simulink model "Aktuator_Klapp"  (R2019b)
settings: Solver=FixedStepAuto  StartTime=0.0  StopTime=9  RelTol=1e-3
values from neighbouring files (symbols this model uses):
  a = 0.047    [Init_Aktuator_Klapp.m]
  Drehzahlkonstante = 1070    [Init_Aktuator.m]    (also in Init_Aktuator_Klapp.m = 569; Init_Aktuator_Steuer.m)
  I_GF = 0.16    [Init_Aktuator_Klapp.m]
  I_Konstante = 20    [Init_Aktuator.m]    (also in Init_Aktuator_Steuer.m)
  I_Motor = 0.0000132    (= 1.32e-05)    [Init_Aktuator_Klapp.m]
  I_Spindel = 0    [Init_Aktuator_Klapp.m]
  Kennliniensteigung = 108*1000    (= 108000)    [Init_Aktuator_Klapp.m]
  M_Hubstange = 0.02    [Init_Aktuator_Klapp.m]
  P_Konstante = 4    [Init_Aktuator.m]    (also in Init_Aktuator_Steuer.m)
  r = 0.016    [Init_Aktuator_Klapp.m]
  Reibungsbeiwert = 0.0018    [Init_Aktuator_Steuer.m]
  Spannung = 12    [Init_Aktuator_Klapp.m]
  Spannung_max = Nennspannung * 2    (= 24)    [Init_Aktuator.m]    (also in Init_Aktuator_Steuer.m = 18)
  Steigung = 27.1*1000    (= 27100)    [Init_Aktuator.m]    (also in Init_Aktuator_Klapp.m = 0.002; Init_Aktuator_Steuer.m)
  Uebersetzung = 200    [Init_Aktuator.m]    (also in Init_Aktuator_Klapp.m = 3.7; Init_Aktuator_Steuer.m)
undefined symbols (not defined in the file or in its folder): Hebelarm, Normalkraft, Wirkungsgrad
libraries: simulink x1
settings Model: Creator=Neu1  LastModifiedBy=Neu1
settings SolverCC: AlgebraicLoopSolver=LineSearch

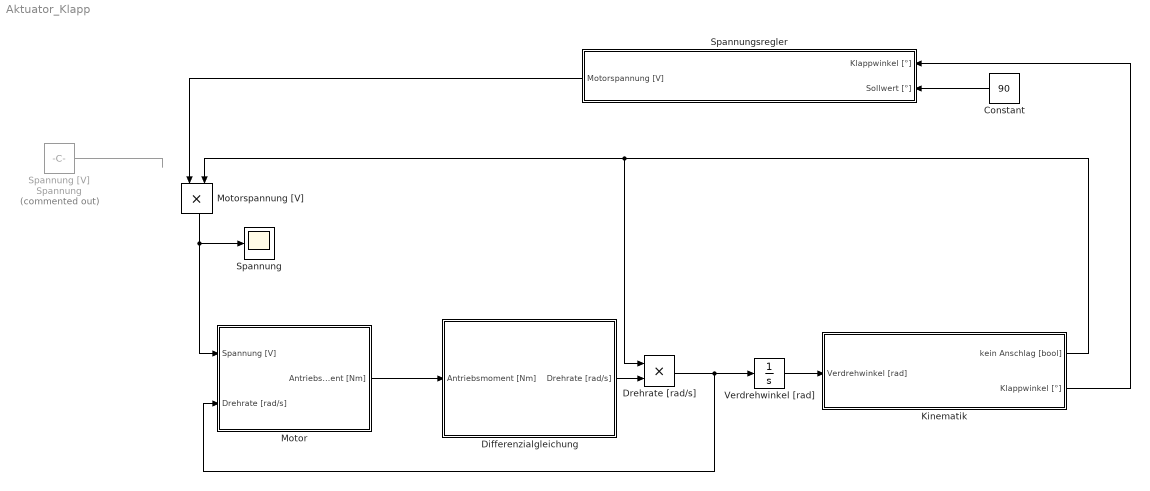
== system Aktuator_Klapp ==
  Constant : Constant  Value=90
  Differenzialgleichung : Subsystem
  Drehrate [rad/s] : Product
  "Kinematik " : Subsystem
  Motor : Subsystem
  Motorspannung [V] : Product
  Spannung : Scope
  Spannung [V] : Constant  Commented=on  Value=Spannung
  Spannungsregler : Subsystem
  Verdrehwinkel [rad] : Integrator
  wires:
  Spannung [V]/1 -> ?
  Drehrate [rad/s]/1 -> Verdrehwinkel [rad]/1, Motor/2(Drehrate [rad/s])
  Motorspannung [V]/1 -> Spannung/1, Motor/1(Spannung [V])
  "Kinematik "/1(kein Anschlag [bool]) -> Motorspannung [V]/2, Drehrate [rad/s]/1
  Motor/1(Antriebsmoment [Nm]) -> Differenzialgleichung/1(Antriebsmoment [Nm])
  Differenzialgleichung/1(Drehrate [rad/s]) -> Drehrate [rad/s]/2
  Verdrehwinkel [rad]/1 -> "Kinematik "/1(Verdrehwinkel [rad])
  "Kinematik "/2(Klappwinkel [°]) -> Spannungsregler/1(Klappwinkel [°])
  Constant/1 -> Spannungsregler/2(Sollwert [°])
  Spannungsregler/1(Motorspannung [V]) -> Motorspannung [V]/1

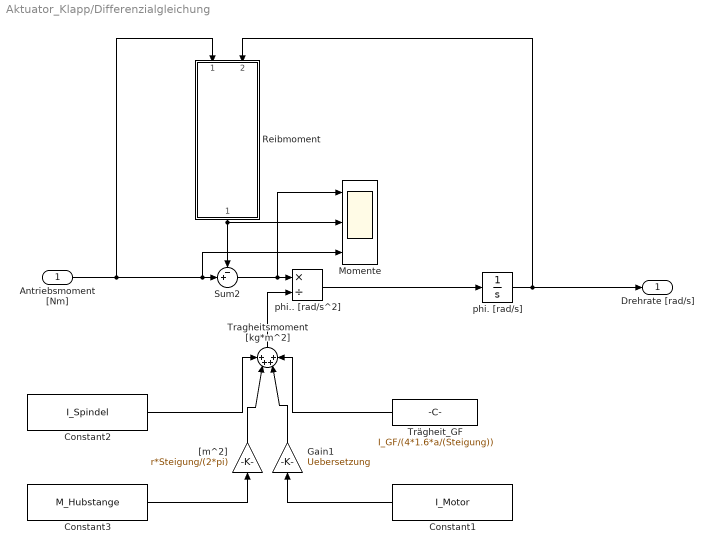
== system Aktuator_Klapp/Differenzialgleichung ==
  Antriebsmoment [Nm] : Inport
  Constant1 : Constant  Value=I_Motor
  Constant2 : Constant  Value=I_Spindel
  Constant3 : Constant  Value=M_Hubstange
  Gain1 : Gain  Gain=Uebersetzung
  Momente : Scope  NumInputPorts=3
  Reibmoment : Subsystem
  Sum2 : Sum  Inputs=-+|
  Tragheitsmoment [kg*m^2] : Sum  Inputs=++++
  Trägheit_GF : Constant  Value=I_GF/(4*1.6*a/(Steigung))  VectorParams1D=off
  "[m^2]" : Gain  Gain=r*Steigung/(2*pi)
  phi. [rad/s] : Integrator
  phi.. [rad/s^2] : Product  Inputs=*/
  Drehrate [rad/s] : Outport
  wires:
  Constant3/1 -> "[m^2]"/1
  Tragheitsmoment [kg*m^2]/1 -> phi.. [rad/s^2]/2
  phi.. [rad/s^2]/1 -> phi. [rad/s]/1
  phi. [rad/s]/1 -> Reibmoment/2(Drehrate [rad/s]), Drehrate [rad/s]/1
  "[m^2]"/1 -> Tragheitsmoment [kg*m^2]/2
  Constant2/1 -> Tragheitsmoment [kg*m^2]/1
  Antriebsmoment [Nm]/1 -> Momente/3, Sum2/2, Reibmoment/1(Antriebsmoment [Nm])
  Constant1/1 -> Gain1/1
  Gain1/1 -> Tragheitsmoment [kg*m^2]/3
  Trägheit_GF/1 -> Tragheitsmoment [kg*m^2]/4
  Sum2/1 -> Momente/1, phi.. [rad/s^2]/1
  Reibmoment/1(Reibmoment [Nm]) -> Momente/2, Sum2/1

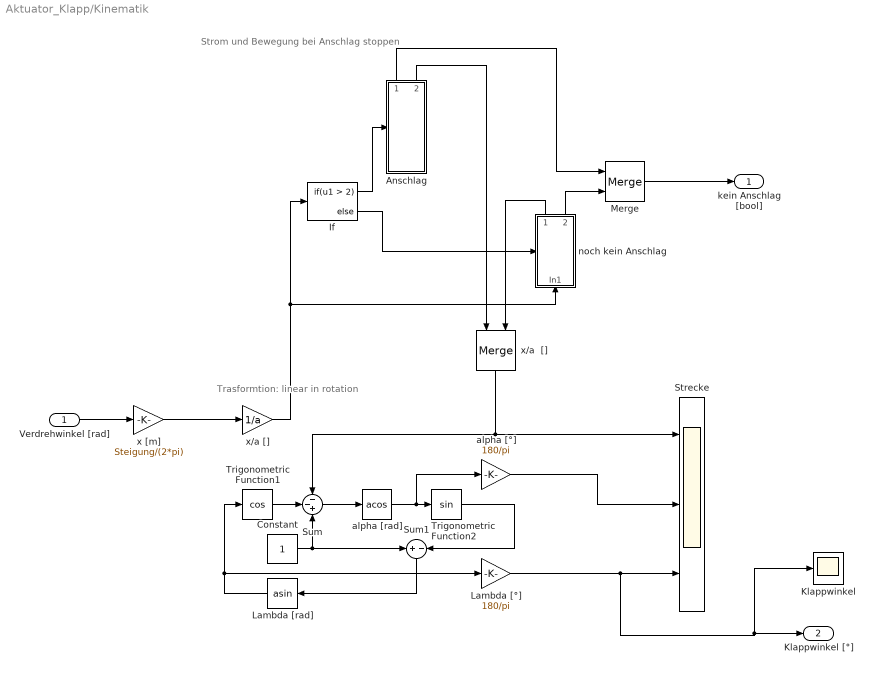
== system Aktuator_Klapp/Kinematik  ==
  note: Strom und Bewegung bei Anschlag stoppen
  note: Trasformtion: linear in rotation
  Verdrehwinkel [rad] : Inport
  Anschlag : Subsystem  TreatAsAtomicUnit=on
  Constant : Constant
  If : If  IfExpression=u1 > 2
  Klappwinkel : Scope
  "Lambda [rad] " : Trigonometry  Operator=asin
  Lambda [°] : Gain  Gain=180/pi
  Merge : Merge
  Strecke : Scope  NumInputPorts=3
  Sum : Sum  Inputs=--+
  Sum1 : Sum  Inputs=+-
  Trigonometric Function1 : Trigonometry  Operator=cos
  Trigonometric Function2 : Trigonometry
  alpha [rad] : Trigonometry  Operator=acos
  alpha [°] : Gain  Gain=180/pi
  noch kein Anschlag : Subsystem  TreatAsAtomicUnit=on
  x [m] : Gain  Gain=Steigung/(2*pi)
  x/a  [] : Merge
  x/a [] : Gain  Gain=1/a
  kein Anschlag [bool] : Outport
  Klappwinkel [°] : Outport  Port=2
  wires:
  Constant/1 -> Sum1/1, Sum/3
  Sum1/1 -> "Lambda [rad] "/1
  Lambda [°]/1 -> Klappwinkel/1, Klappwinkel [°]/1, Strecke/3
  Trigonometric Function2/1 -> Sum1/2
  x/a []/1 -> If/1, noch kein Anschlag/1(In1)
  Anschlag/1(Out1) -> Merge/1
  alpha [°]/1 -> Strecke/2
  If/1 -> Anschlag/Action
  If/2 -> noch kein Anschlag/Action
  alpha [rad]/1 -> alpha [°]/1, Trigonometric Function2/1
  "Lambda [rad] "/1 -> Trigonometric Function1/1, Lambda [°]/1
  Trigonometric Function1/1 -> Sum/2
  Sum/1 -> alpha [rad]/1
  Merge/1 -> kein Anschlag [bool]/1
  noch kein Anschlag/2(Out1) -> Merge/2
  Verdrehwinkel [rad]/1 -> x [m]/1
  x [m]/1 -> x/a []/1
  noch kein Anschlag/1(Out2) -> x/a  []/2
  Anschlag/2(Out2) -> x/a  []/1
  x/a  []/1 -> Strecke/1, Sum/1

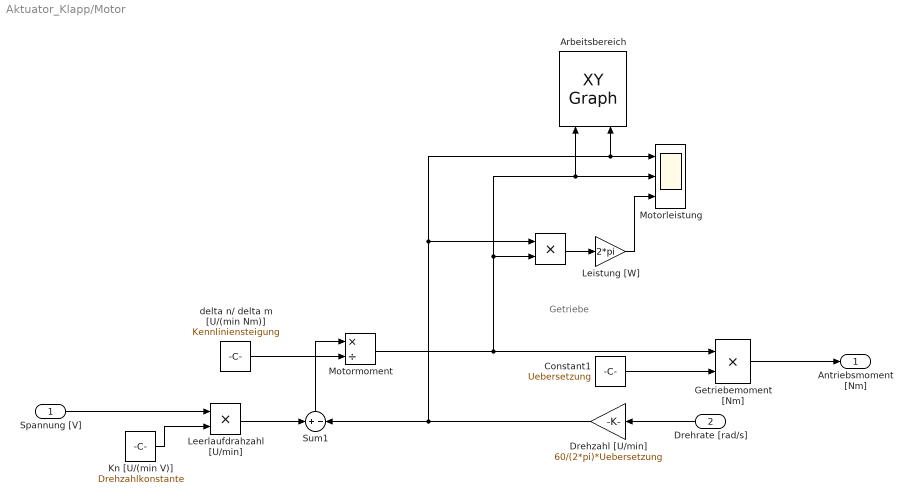
== system Aktuator_Klapp/Motor ==
  note: Getriebe
  Spannung [V] : Inport
  Drehrate [rad/s] : Inport  Port=2
  " " : Product
  "Arbeitsbereich " : simulink/Sinks/XY Graph  xmin=-0.01  xmax=0.07  ymin=-1000  ymax=6000  st=0.1
  Constant1 : Constant  Value=Uebersetzung
  Drehzahl [U/min] : Gain  Gain=60/(2*pi)*Uebersetzung
  Getriebemoment [Nm] : Product
  Kn [U/(min V)] : Constant  Value=Drehzahlkonstante
  Leerlaufdrahzahl [U/min] : Product
  Leistung [W] : Gain  Gain=2*pi
  Motorleistung : Scope  NumInputPorts=3
  Motormoment : Product  Inputs=*/
  Sum1 : Sum  Inputs=+|-
  delta n/ delta m [U/(min Nm)] : Constant  Value=Kennliniensteigung
  Antriebsmoment [Nm] : Outport
  wires:
  delta n/ delta m [U/(min Nm)]/1 -> Motormoment/2
  Sum1/1 -> Motormoment/1
  Motormoment/1 -> Getriebemoment [Nm]/1, Motorleistung/2, "Arbeitsbereich "/1, " "/2
  Spannung [V]/1 -> Leerlaufdrahzahl [U/min]/1
  Leerlaufdrahzahl [U/min]/1 -> Sum1/1
  Kn [U/(min V)]/1 -> Leerlaufdrahzahl [U/min]/2
  Drehzahl [U/min]/1 -> Motorleistung/1, "Arbeitsbereich "/2, " "/1, Sum1/2
  Constant1/1 -> Getriebemoment [Nm]/2
  Getriebemoment [Nm]/1 -> Antriebsmoment [Nm]/1
  Drehrate [rad/s]/1 -> Drehzahl [U/min]/1
  " "/1 -> Leistung [W]/1
  Leistung [W]/1 -> Motorleistung/3

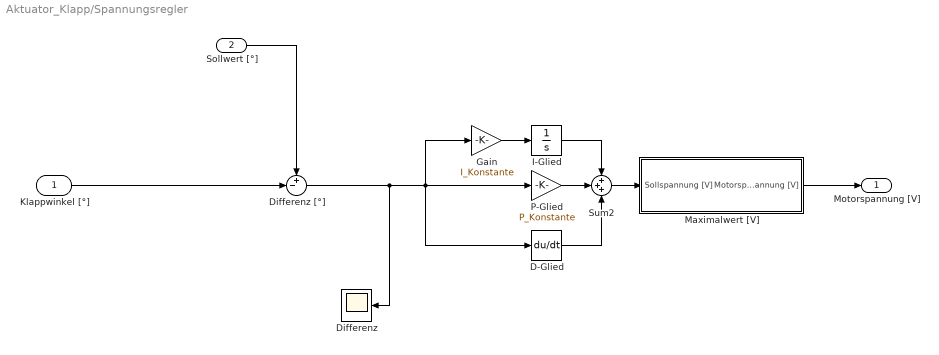
== system Aktuator_Klapp/Spannungsregler ==
  Klappwinkel [°] : Inport
  Sollwert [°] : Inport  Port=2
  D-Glied : Derivative  CoefficientInTFapproximation=D_Konstante
  Differenz : Scope
  Differenz [°] : Sum  Inputs=+-|
  Gain : Gain  Gain=I_Konstante
  I-Glied : Integrator
  Maximalwert [V] : Subsystem
  P-Glied : Gain  Gain=P_Konstante
  Sum2 : Sum  Inputs=+++
  Motorspannung [V] : Outport
  wires:
  Sum2/1 -> Maximalwert [V]/1("Sollspannung [V] ")
  Gain/1 -> I-Glied/1
  D-Glied/1 -> Sum2/3
  Differenz [°]/1 -> Gain/1, P-Glied/1, D-Glied/1, Differenz/1
  P-Glied/1 -> Sum2/2
  Sollwert [°]/1 -> Differenz [°]/1
  I-Glied/1 -> Sum2/1
  Klappwinkel [°]/1 -> Differenz [°]/2
  Maximalwert [V]/1("Motorspannung [V] ") -> Motorspannung [V]/1

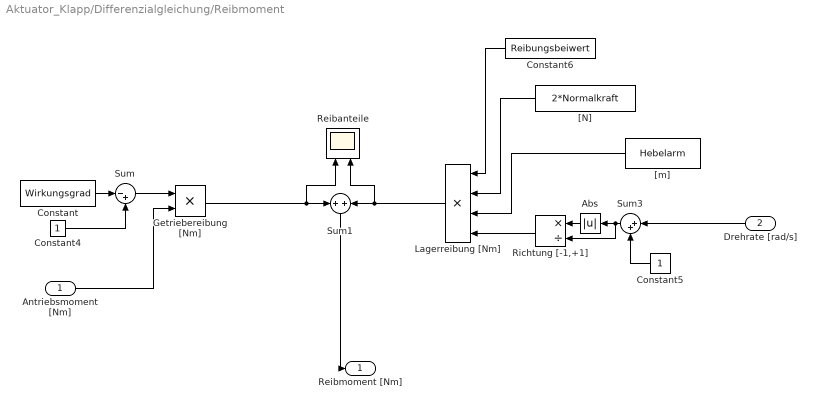
== system Aktuator_Klapp/Differenzialgleichung/Reibmoment ==
  Antriebsmoment [Nm] : Inport
  Drehrate [rad/s] : Inport  Port=2
  Abs : Abs
  Constant : Constant  Value=Wirkungsgrad
  Constant4 : Constant
  Constant5 : Constant
  Constant6 : Constant  Value=Reibungsbeiwert
  Getriebereibung [Nm] : Product
  Lagerreibung [Nm] : Product  Inputs=4
  Reibanteile : Scope  NumInputPorts=2
  Richtung [-1,+1] : Product  Inputs=*/
  Sum : Sum  Inputs=|-+
  Sum1 : Sum  Inputs=+|+
  Sum3 : Sum  Inputs=|++
  "[N]" : Constant  Value=2*Normalkraft
  "[m]" : Constant  Value=Hebelarm
  Reibmoment [Nm] : Outport
  wires:
  Antriebsmoment [Nm]/1 -> Getriebereibung [Nm]/2
  Sum/1 -> Getriebereibung [Nm]/1
  Constant4/1 -> Sum/2
  Getriebereibung [Nm]/1 -> Reibanteile/1, Sum1/1
  Sum3/1 -> Richtung [-1,+1]/2, Abs/1
  Constant5/1 -> Sum3/2
  Constant6/1 -> Lagerreibung [Nm]/1
  Constant/1 -> Sum/1
  "[N]"/1 -> Lagerreibung [Nm]/2
  Lagerreibung [Nm]/1 -> Reibanteile/2, Sum1/2
  Abs/1 -> Richtung [-1,+1]/1
  Richtung [-1,+1]/1 -> Lagerreibung [Nm]/4
  Sum1/1 -> Reibmoment [Nm]/1
  Drehrate [rad/s]/1 -> Sum3/1
  "[m]"/1 -> Lagerreibung [Nm]/3

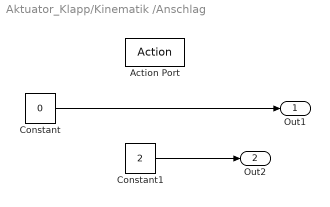
== system Aktuator_Klapp/Kinematik /Anschlag ==
  Action Port : ActionPort  ActionPortLabel=if(u1 > 2)
  Constant : Constant  Value=0
  Constant1 : Constant  Value=2
  Out1 : Outport
  Out2 : Outport  Port=2
  wires:
  Constant/1 -> Out1/1
  Constant1/1 -> Out2/1

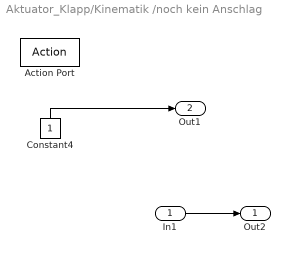
== system Aktuator_Klapp/Kinematik /noch kein Anschlag ==
  In1 : Inport
  Action Port : ActionPort  ActionPortLabel=else
  Constant4 : Constant
  Out2 : Outport
  Out1 : Outport  Port=2
  wires:
  Constant4/1 -> Out1/1
  In1/1 -> Out2/1

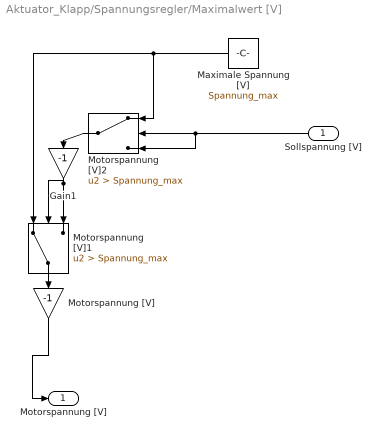
== system Aktuator_Klapp/Spannungsregler/Maximalwert [V] ==
  "Sollspannung [V] " : Inport
  Gain1 : Gain  Gain=-1
  Maximale Spannung [V] : Constant  Value=Spannung_max
  Motorspannung [V] : Gain  Gain=-1
  Motorspannung [V]1 : Switch  Criteria=u2 > Threshold  Threshold=Spannung_max
  Motorspannung [V]2 : Switch  Criteria=u2 > Threshold  Threshold=Spannung_max
  "Motorspannung [V] " : Outport
  wires:
  Motorspannung [V]2/1 -> Gain1/1
  Gain1/1 -> Motorspannung [V]1/2, Motorspannung [V]1/3
  "Sollspannung [V] "/1 -> Motorspannung [V]2/3, Motorspannung [V]2/2
  Maximale Spannung [V]/1 -> Motorspannung [V]1/1, Motorspannung [V]2/1
  Motorspannung [V]1/1 -> Motorspannung [V]/1
  Motorspannung [V]/1 -> "Motorspannung [V] "/1
